simulink model "verify_microCHP_constant_mdl"  (R2016b)
settings: Solver=ode45  StartTime=0  StopTime=3*3600  MaxStep=60  RelTol=1e-3  EnableMultiTasking=on
libraries: carnot x3
settings Model: Creator=drhf  LastModifiedBy=drhf
settings DataIOCC: SaveFormat=Array  SignalLoggingSaveFormat=ModelDataLogs
settings OptimizationCC: ExpressionDepthLimit=2147483647  LifeSpan=inf
settings DebuggingCC: UnderspecifiedInitializationDetection=Classic  MergeDetectMultiDrivingBlocksExec=none  SolverPrmCheckMsg=warning  FcnCallInpInsideContextMsg=warning  StateNameClashWarn=warning  SFUnexpectedBacktrackingDiag=warning  SFNoUnconditionalDefaultTransitionDiag=warning  SFExecutionAtInitializationDiag=none
settings HardwareCC: ProdBitPerPointer=32  ProdBitPerSizeT=32  ProdBitPerPtrDiffT=32  ProdLargestAtomicFloat=None  ProdIntDivRoundTo=Undefined  ProdEndianess=Unspecified  ProdWordSize=32  ProdHWDeviceType=32-bit Generic
settings ModelReferenceCC: PropagateSignalLabelsOutOfModel=off
settings GRTTargetCC: TargetLangStandard=C89/C90 (ANSI)  GeneratePreprocessorConditionals=Disable all  CombineOutputUpdateFcns=off  GRTInterface=on
settings ConfigComp: CovMetricSettings=dw  CovHtmlReporting=on  CovSaveCumulativeToWorkspaceVar=on  CovSaveSingleToWorkspaceVar=on  CovExternalEMLEnable=off

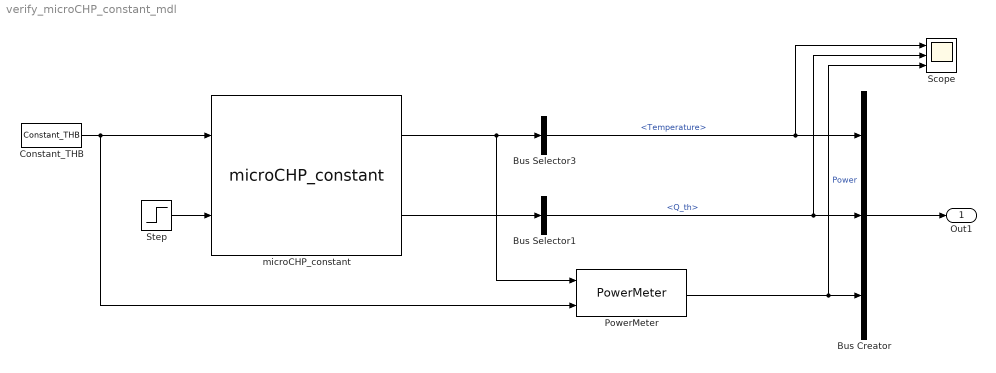
== system verify_microCHP_constant_mdl ==
  Bus Creator : BusCreator  Inputs=3
  Bus Selector1 : BusSelector  OutputSignals=Q_th
  Bus Selector3 : BusSelector  OutputSignals=Temperature
  Constant_THB : carnot/Source/Simple/Constant_THB  t=60  mdot=1500/3600  p=1e5  mID=No Pressure Drop  fluid=Water  mix=0  mix2=0  mix3=0  dia=0.02  hgt=0
  PowerMeter : carnot/Control/PowerMeter
  Scope : Scope  NumInputPorts=3
  Step : Step  Time=3600  SampleTime=0
  microCHP_constant : carnot/Source/Cogeneration/microCHP_constant  P_th=11520  P_el=5500  P_fuel=22030  T_flow_setpoint=80  T_return_max=75
  Out1 : Outport
  wires:
  Bus Selector3/1 -> Scope/1, Bus Creator/1  "<Temperature>"
  Constant_THB/1 -> PowerMeter/2, microCHP_constant/1
  Step/1 -> microCHP_constant/2
  microCHP_constant/1 -> PowerMeter/1, Bus Selector3/1
  microCHP_constant/2 -> Bus Selector1/1
  Bus Creator/1 -> Out1/1
  PowerMeter/1 -> Scope/3, Bus Creator/3  "Power"
  Bus Selector1/1 -> Scope/2, Bus Creator/2  "<Q_th>"
